simulink model "IEEE_13_BUS_Radial"  (R2021b)
settings: Solver=VariableStepAuto  StartTime=0.0  StopTime=48  RelTol=1e-3
undefined symbols (not defined in the file or in its folder): f611, f632, f633, f634, f645, f646, f650, f652, f671, f675, f680, f684, f692
libraries: simulink x416, slpidlib x13
(part 5 of 7)

== system IEEE_13_BUS_Radial/f692/PCU ==
  m : Inport
  setup : Inport  Port=2
  Psp : Inport  Port=3
  Bus Creator : BusCreator  Inputs=1
  Demux : Demux  Outputs=[1 -1]
  Mux2 : Mux  Inputs=16
  PID Controller : slpidlib/PID Controller  Controller=PID  Form=Parallel  TimeDomain=Continuous-time  UseExternalTs=off  SampleTime=-1  IntegratorMethod=Forward Euler  FilterMethod=Forward Euler  ControllerParametersSource=internal  P=80  I=20  D=10  UseFilter=on  N=100  TunerSelectOption=Transfer Function Based (PID Tuner App)  InitialConditionSource=internal  InitialConditionForIntegrator=0  InitialConditionForFilter=0  DifferentiatorICPrevScaledInput=0  ExternalReset=none  TrackingMode=off  Kt=1  LimitOutput=off  SatLimitsSource=internal  UpperSaturationLimit=inf  LowerSaturationLimit=-inf  LinearizeAsGain=on  AntiWindupMode=none  Kb=1  POutMin=[]  POutMax=[]  IOutMin=[]  IOutMax=[]  DOutMin=[]  DOutMax=[]  NOutMin=[]  NOutMax=[]  SumOutMin=[]  SumOutMax=[]  SaturationOutMin=[]  SaturationOutMax=[]  PParamMin=[]  PParamMax=[]  IParamMin=[]  IParamMax=[]  DParamMin=[]  DParamMax=[]  NParamMin=[]  NParamMax=[]  KbParamMin=[]  KbParamMax=[]  KtParamMin=[]  KtParamMax=[]  KbOutMin=[]  KbOutMax=[]  KtOutMin=[]  KtOutMax=[]  IntegratorOutMin=[]  IntegratorOutMax=[]  FilterOutMin=[]  FilterOutMax=[]  SumI1OutMin=[]  SumI1OutMax=[]  SumI2OutMin=[]  SumI2OutMax=[]  SumI3OutMin=[]  SumI3OutMax=[]  SumI4OutMin=[]  SumI4OutMax=[]  SumDOutMin=[]  SumDOutMax=[]  DifferentiatorOutMin=[]  DifferentiatorOutMax=[]  FilterDiffOutCoefMin=[]  FilterDiffOutCoefMax=[]  ReciprocalOutMin=[]  ReciprocalOutMax=[]  SumDenOutMin=[]  SumDenOutMax=[]  SumNumOutMin=[]  SumNumOutMax=[]  DivideOutMin=[]  DivideOutMax=[]  UdiffTsProdOutMin=[]  UdiffTsProdOutMax=[]  NTsProdOutMin=[]  NTsProdOutMax=[]  UintegralTsProdOutMin=[]  UintegralTsProdOutMax=[]  UngainTsProdOutMin=[]  UngainTsProdOutMax=[]  IntegratorContinuousStateAttributes=''  IntegratorStateMustResolveToSignalObject=off  IntegratorRTWStateStorageClass=Auto  FilterContinuousStateAttributes=''  FilterStateMustResolveToSignalObject=off  FilterRTWStateStorageClass=Auto  ParallelPVariant=InternalParameters  IdealPVariant=Disabled  IVariant=InternalParameters  DVariant=InternalParameters  IntegratorVariant=Continuous  SatVariant=Disabled  AWVariant=Passthrough  PCopyVariant=Disabled  TRVariant=Disabled  FdbkBlocksVariant=Forward  IdealPFdbkVariant=Disabled  SatFdbkVariant=Disabled  DerivativeFilterVariant=ContFilter  NVariant=InternalParameters  NCopyVariant=Disabled  FilterICVariant=InternalICsFilter  IntegratorICVariant=InternalICs  ExternalResetVariant=Disabled  TRSumVariant=Passthrough  SumFdbkVariant=Disabled  SumVariant=Sum_PID  TsampFilterVariant=InternalTs  TsampNgainVariant=Passthrough  TsampIntegralVariant=Passthrough  ExternalSaturationOutDataTypeStr=Inherit: Same as second input
  Sum : Sum  Inputs=+-
  Terminator : Terminator
  Terminator1 : Terminator
  sPCC : Constant  Value=0
  sPoLC{1,3..16} (15 alike) : Constant  Value=0
  sPoLC2 : Constant
  PCCctrl : Outport  VectorParamsAs1DForOutWhenUnconnected=off
  PoLCctrl : Outport  Port=2  VectorParamsAs1DForOutWhenUnconnected=off
  DEVctrl : Outport  Port=3  VectorParamsAs1DForOutWhenUnconnected=off
  wires:
  sPoLC8/1 -> Mux2/8
  sPoLC11/1 -> Mux2/11
  sPoLC4/1 -> Mux2/4
  sPoLC16/1 -> Mux2/16
  sPoLC14/1 -> Mux2/14
  sPoLC10/1 -> Mux2/10
  sPoLC12/1 -> Mux2/12
  sPoLC1/1 -> Mux2/1
  sPoLC15/1 -> Mux2/15
  sPoLC6/1 -> Mux2/6
  sPoLC13/1 -> Mux2/13
  sPoLC7/1 -> Mux2/7
  sPoLC9/1 -> Mux2/9
  sPoLC2/1 -> Mux2/2
  sPoLC3/1 -> Mux2/3
  sPoLC5/1 -> Mux2/5
  Mux2/1 -> PoLCctrl/1
  sPCC/1 -> PCCctrl/1
  setup/1 -> Terminator/1
  Psp/1 -> Sum/1
  Bus Creator/1 -> DEVctrl/1
  m/1 -> Demux/1
  Demux/1 -> Sum/2
  Sum/1 -> PID Controller/1
  PID Controller/1 -> Bus Creator/1  "pidCV"
  Demux/2 -> Terminator1/1

== system IEEE_13_BUS_Radial/f692/SYSTEM_INTERFACE ==
  ctrl : Inport
  devices : Inport  Port=2
  e_PoLC1 : Inport  Port=3
  e_PoLC2 : Inport  Port=4
  e_PoLC3 : Inport  Port=5
  e_PoLC4 : Inport  Port=6
  e_PoLC5 : Inport  Port=7
  e_PoLC6 : Inport  Port=8
  e_PoLC7 : Inport  Port=9
  e_PoLC8 : Inport  Port=10
  e_PoLC9 : Inport  Port=11
  e_PoLC10 : Inport  Port=12
  e_PoLC11 : Inport  Port=13
  e_PoLC12 : Inport  Port=14
  e_PoLC13 : Inport  Port=15
  e_PoLC14 : Inport  Port=16
  e_PoLC15 : Inport  Port=17
  e_PoLC16 : Inport  Port=18
  Demux : Demux  Outputs=16
  Demux1 : Demux  Outputs=16
  S PoLC{1..16} (16 alike) : Switch  Criteria=u2 > Threshold
  PoLC1 : Outport  VectorParamsAs1DForOutWhenUnconnected=off
  PoLC2 : Outport  Port=2  VectorParamsAs1DForOutWhenUnconnected=off
  PoLC3 : Outport  Port=3  VectorParamsAs1DForOutWhenUnconnected=off
  PoLC4 : Outport  Port=4  VectorParamsAs1DForOutWhenUnconnected=off
  PoLC5 : Outport  Port=5  VectorParamsAs1DForOutWhenUnconnected=off
  PoLC6 : Outport  Port=6  VectorParamsAs1DForOutWhenUnconnected=off
  PoLC7 : Outport  Port=7  VectorParamsAs1DForOutWhenUnconnected=off
  PoLC8 : Outport  Port=8  VectorParamsAs1DForOutWhenUnconnected=off
  PoLC9 : Outport  Port=9  VectorParamsAs1DForOutWhenUnconnected=off
  PoLC10 : Outport  Port=10  VectorParamsAs1DForOutWhenUnconnected=off
  PoLC11 : Outport  Port=11  VectorParamsAs1DForOutWhenUnconnected=off
  PoLC12 : Outport  Port=12  VectorParamsAs1DForOutWhenUnconnected=off
  PoLC13 : Outport  Port=13  VectorParamsAs1DForOutWhenUnconnected=off
  PoLC14 : Outport  Port=14  VectorParamsAs1DForOutWhenUnconnected=off
  PoLC15 : Outport  Port=15  VectorParamsAs1DForOutWhenUnconnected=off
  PoLC16 : Outport  Port=16  VectorParamsAs1DForOutWhenUnconnected=off
  wires:
  S PoLC9/1 -> PoLC9/1
  e_PoLC4/1 -> S PoLC4/3
  e_PoLC11/1 -> S PoLC11/3
  S PoLC16/1 -> PoLC16/1
  e_PoLC8/1 -> S PoLC8/3
  S PoLC6/1 -> PoLC6/1
  e_PoLC7/1 -> S PoLC7/3
  S PoLC13/1 -> PoLC13/1
  e_PoLC5/1 -> S PoLC5/3
  S PoLC10/1 -> PoLC10/1
  e_PoLC9/1 -> S PoLC9/3
  e_PoLC12/1 -> S PoLC12/3
  e_PoLC6/1 -> S PoLC6/3
  S PoLC15/1 -> PoLC15/1
  S PoLC1/1 -> PoLC1/1
  S PoLC12/1 -> PoLC12/1
  S PoLC11/1 -> PoLC11/1
  e_PoLC14/1 -> S PoLC14/3
  e_PoLC10/1 -> S PoLC10/3
  S PoLC5/1 -> PoLC5/1
  e_PoLC1/1 -> S PoLC1/3
  e_PoLC15/1 -> S PoLC15/3
  e_PoLC16/1 -> S PoLC16/3
  S PoLC7/1 -> PoLC7/1
  e_PoLC3/1 -> S PoLC3/3
  e_PoLC13/1 -> S PoLC13/3
  S PoLC8/1 -> PoLC8/1
  e_PoLC2/1 -> S PoLC2/3
  S PoLC4/1 -> PoLC4/1
  S PoLC2/1 -> PoLC2/1
  S PoLC14/1 -> PoLC14/1
  S PoLC3/1 -> PoLC3/1
  ctrl/1 -> Demux/1
  Demux/1 -> S PoLC1/2
  Demux/2 -> S PoLC2/2
  Demux/3 -> S PoLC3/2
  Demux/4 -> S PoLC4/2
  Demux/5 -> S PoLC5/2
  Demux/6 -> S PoLC6/2
  Demux/7 -> S PoLC7/2
  Demux/8 -> S PoLC8/2
  Demux/9 -> S PoLC9/2
  Demux/10 -> S PoLC10/2
  Demux/11 -> S PoLC11/2
  Demux/12 -> S PoLC12/2
  Demux/13 -> S PoLC13/2
  Demux/14 -> S PoLC14/2
  Demux/15 -> S PoLC15/2
  Demux/16 -> S PoLC16/2
  devices/1 -> Demux1/1
  Demux1/1 -> S PoLC1/1
  Demux1/2 -> S PoLC2/1
  Demux1/3 -> S PoLC3/1
  Demux1/4 -> S PoLC4/1
  Demux1/5 -> S PoLC5/1
  Demux1/6 -> S PoLC6/1
  Demux1/7 -> S PoLC7/1
  Demux1/8 -> S PoLC8/1
  Demux1/9 -> S PoLC9/1
  Demux1/10 -> S PoLC10/1
  Demux1/11 -> S PoLC11/1
  Demux1/12 -> S PoLC12/1
  Demux1/13 -> S PoLC13/1
  Demux1/14 -> S PoLC14/1
  Demux1/15 -> S PoLC15/1
  Demux1/16 -> S PoLC16/1

== system IEEE_13_BUS_Radial/f611/CONTROLLERS/lPoLC1 ==
  Sum : Sum  Inputs=|++
  base : simulink/Sources/Repeating Sequence Stair  OutValues=f611.PoLC1.l  tsamp=f611.PoLC1.ST  OutMin=[]  OutMax=[]  OutDataTypeStr=double  OutputDataTypeScalingMode=double  OutDataType=fixdt(0,8)  ConRadixGroup=Best Precision: Vector-wise  OutScaling=2^-12
  noise : simulink/Sources/Band-Limited White Noise  Cov=f611.PoLC1.Noise  Ts=f611.PoLC1.NoiseST  seed=f611.PoLC1.NoiseSD
  P : Outport  VectorParamsAs1DForOutWhenUnconnected=off
  wires:
  Sum/1 -> P/1
  noise/1 -> Sum/2
  base/1 -> Sum/1

== system IEEE_13_BUS_Radial/f611/CONTROLLERS/lPoLC10 ==
  Sum : Sum  Inputs=|++
  base : simulink/Sources/Repeating Sequence Stair  OutValues=f611.PoLC10.l  tsamp=f611.PoLC10.ST  OutMin=[]  OutMax=[]  OutDataTypeStr=double  OutputDataTypeScalingMode=double  OutDataType=fixdt(0,8)  ConRadixGroup=Best Precision: Vector-wise  OutScaling=2^-12
  noise : simulink/Sources/Band-Limited White Noise  Cov=f611.PoLC10.Noise  Ts=f611.PoLC10.NoiseST  seed=f611.PoLC10.NoiseSD
  P : Outport  VectorParamsAs1DForOutWhenUnconnected=off
  wires:
  Sum/1 -> P/1
  noise/1 -> Sum/2
  base/1 -> Sum/1

== system IEEE_13_BUS_Radial/f611/CONTROLLERS/lPoLC11 ==
  Sum : Sum  Inputs=|++
  base : simulink/Sources/Repeating Sequence Stair  OutValues=f611.PoLC11.l  tsamp=f611.PoLC11.ST  OutMin=[]  OutMax=[]  OutDataTypeStr=double  OutputDataTypeScalingMode=double  OutDataType=fixdt(0,8)  ConRadixGroup=Best Precision: Vector-wise  OutScaling=2^-12
  noise : simulink/Sources/Band-Limited White Noise  Cov=f611.PoLC11.Noise  Ts=f611.PoLC11.NoiseST  seed=f611.PoLC11.NoiseSD
  P : Outport  VectorParamsAs1DForOutWhenUnconnected=off
  wires:
  Sum/1 -> P/1
  noise/1 -> Sum/2
  base/1 -> Sum/1

== system IEEE_13_BUS_Radial/f611/CONTROLLERS/lPoLC12 ==
  Sum : Sum  Inputs=|++
  base : simulink/Sources/Repeating Sequence Stair  OutValues=f611.PoLC12.l  tsamp=f611.PoLC12.ST  OutMin=[]  OutMax=[]  OutDataTypeStr=double  OutputDataTypeScalingMode=double  OutDataType=fixdt(0,8)  ConRadixGroup=Best Precision: Vector-wise  OutScaling=2^-12
  noise : simulink/Sources/Band-Limited White Noise  Cov=f611.PoLC12.Noise  Ts=f611.PoLC12.NoiseST  seed=f611.PoLC12.NoiseSD
  P : Outport  VectorParamsAs1DForOutWhenUnconnected=off
  wires:
  Sum/1 -> P/1
  noise/1 -> Sum/2
  base/1 -> Sum/1

== system IEEE_13_BUS_Radial/f611/CONTROLLERS/lPoLC13 ==
  Sum : Sum  Inputs=|++
  base : simulink/Sources/Repeating Sequence Stair  OutValues=f611.PoLC13.l  tsamp=f611.PoLC13.ST  OutMin=[]  OutMax=[]  OutDataTypeStr=double  OutputDataTypeScalingMode=double  OutDataType=fixdt(0,8)  ConRadixGroup=Best Precision: Vector-wise  OutScaling=2^-12
  noise : simulink/Sources/Band-Limited White Noise  Cov=f611.PoLC13.Noise  Ts=f611.PoLC13.NoiseST  seed=f611.PoLC13.NoiseSD
  P : Outport  VectorParamsAs1DForOutWhenUnconnected=off
  wires:
  Sum/1 -> P/1
  noise/1 -> Sum/2
  base/1 -> Sum/1

== system IEEE_13_BUS_Radial/f611/CONTROLLERS/lPoLC14 ==
  Sum : Sum  Inputs=|++
  base : simulink/Sources/Repeating Sequence Stair  OutValues=f611.PoLC14.l  tsamp=f611.PoLC14.ST  OutMin=[]  OutMax=[]  OutDataTypeStr=double  OutputDataTypeScalingMode=double  OutDataType=fixdt(0,8)  ConRadixGroup=Best Precision: Vector-wise  OutScaling=2^-12
  noise : simulink/Sources/Band-Limited White Noise  Cov=f611.PoLC14.Noise  Ts=f611.PoLC14.NoiseST  seed=f611.PoLC14.NoiseSD
  P : Outport  VectorParamsAs1DForOutWhenUnconnected=off
  wires:
  Sum/1 -> P/1
  noise/1 -> Sum/2
  base/1 -> Sum/1

== system IEEE_13_BUS_Radial/f611/CONTROLLERS/lPoLC15 ==
  Sum : Sum  Inputs=|++
  base : simulink/Sources/Repeating Sequence Stair  OutValues=f611.PoLC15.l  tsamp=f611.PoLC15.ST  OutMin=[]  OutMax=[]  OutDataTypeStr=double  OutputDataTypeScalingMode=double  OutDataType=fixdt(0,8)  ConRadixGroup=Best Precision: Vector-wise  OutScaling=2^-12
  noise : simulink/Sources/Band-Limited White Noise  Cov=f611.PoLC15.Noise  Ts=f611.PoLC15.NoiseST  seed=f611.PoLC15.NoiseSD
  P : Outport  VectorParamsAs1DForOutWhenUnconnected=off
  wires:
  Sum/1 -> P/1
  noise/1 -> Sum/2
  base/1 -> Sum/1

== system IEEE_13_BUS_Radial/f611/CONTROLLERS/lPoLC16 ==
  cv : Inport
  Sum : Sum  Inputs=|++
  Terminator : Terminator
  base : simulink/Sources/Repeating Sequence Stair  OutValues=f611.PoLC16.l  tsamp=f611.PoLC16.ST  OutMin=[]  OutMax=[]  OutDataTypeStr=double  OutputDataTypeScalingMode=double  OutDataType=fixdt(0,8)  ConRadixGroup=Best Precision: Vector-wise  OutScaling=2^-12
  noise : simulink/Sources/Band-Limited White Noise  Cov=f611.PoLC16.Noise  Ts=f611.PoLC16.NoiseST  seed=f611.PoLC16.NoiseSD
  P : Outport  VectorParamsAs1DForOutWhenUnconnected=off
  wires:
  Sum/1 -> Terminator/1
  noise/1 -> Sum/2
  base/1 -> Sum/1
  cv/1 -> P/1

== system IEEE_13_BUS_Radial/f611/CONTROLLERS/lPoLC2 ==
  Sum : Sum  Inputs=|++
  base : simulink/Sources/Repeating Sequence Stair  OutValues=f611.PoLC2.l  tsamp=f611.PoLC2.ST  OutMin=[]  OutMax=[]  OutDataTypeStr=double  OutputDataTypeScalingMode=double  OutDataType=fixdt(0,8)  ConRadixGroup=Best Precision: Vector-wise  OutScaling=2^-12
  noise : simulink/Sources/Band-Limited White Noise  Cov=f611.PoLC2.Noise  Ts=f611.PoLC2.NoiseST  seed=f611.PoLC2.NoiseSD
  P : Outport  VectorParamsAs1DForOutWhenUnconnected=off
  wires:
  Sum/1 -> P/1
  noise/1 -> Sum/2
  base/1 -> Sum/1

== system IEEE_13_BUS_Radial/f611/CONTROLLERS/lPoLC3 ==
  Sum : Sum  Inputs=|++
  base : simulink/Sources/Repeating Sequence Stair  OutValues=f611.PoLC3.l  tsamp=f611.PoLC3.ST  OutMin=[]  OutMax=[]  OutDataTypeStr=double  OutputDataTypeScalingMode=double  OutDataType=fixdt(0,8)  ConRadixGroup=Best Precision: Vector-wise  OutScaling=2^-12
  noise : simulink/Sources/Band-Limited White Noise  Cov=f611.PoLC3.Noise  Ts=f611.PoLC3.NoiseST  seed=f611.PoLC3.NoiseSD
  P : Outport  VectorParamsAs1DForOutWhenUnconnected=off
  wires:
  Sum/1 -> P/1
  noise/1 -> Sum/2
  base/1 -> Sum/1

== system IEEE_13_BUS_Radial/f611/CONTROLLERS/lPoLC4 ==
  Sum : Sum  Inputs=|++
  base : simulink/Sources/Repeating Sequence Stair  OutValues=f611.PoLC4.l  tsamp=f611.PoLC4.ST  OutMin=[]  OutMax=[]  OutDataTypeStr=double  OutputDataTypeScalingMode=double  OutDataType=fixdt(0,8)  ConRadixGroup=Best Precision: Vector-wise  OutScaling=2^-12
  noise : simulink/Sources/Band-Limited White Noise  Cov=f611.PoLC4.Noise  Ts=f611.PoLC4.NoiseST  seed=f611.PoLC4.NoiseSD
  P : Outport  VectorParamsAs1DForOutWhenUnconnected=off
  wires:
  Sum/1 -> P/1
  noise/1 -> Sum/2
  base/1 -> Sum/1

== system IEEE_13_BUS_Radial/f611/CONTROLLERS/lPoLC5 ==
  Sum : Sum  Inputs=|++
  base : simulink/Sources/Repeating Sequence Stair  OutValues=f611.PoLC5.l  tsamp=f611.PoLC5.ST  OutMin=[]  OutMax=[]  OutDataTypeStr=double  OutputDataTypeScalingMode=double  OutDataType=fixdt(0,8)  ConRadixGroup=Best Precision: Vector-wise  OutScaling=2^-12
  noise : simulink/Sources/Band-Limited White Noise  Cov=f611.PoLC5.Noise  Ts=f611.PoLC5.NoiseST  seed=f611.PoLC5.NoiseSD
  P : Outport  VectorParamsAs1DForOutWhenUnconnected=off
  wires:
  Sum/1 -> P/1
  noise/1 -> Sum/2
  base/1 -> Sum/1

== system IEEE_13_BUS_Radial/f611/CONTROLLERS/lPoLC6 ==
  Sum : Sum  Inputs=|++
  base : simulink/Sources/Repeating Sequence Stair  OutValues=f611.PoLC6.l  tsamp=f611.PoLC6.ST  OutMin=[]  OutMax=[]  OutDataTypeStr=double  OutputDataTypeScalingMode=double  OutDataType=fixdt(0,8)  ConRadixGroup=Best Precision: Vector-wise  OutScaling=2^-12
  noise : simulink/Sources/Band-Limited White Noise  Cov=f611.PoLC6.Noise  Ts=f611.PoLC6.NoiseST  seed=f611.PoLC6.NoiseSD
  P : Outport  VectorParamsAs1DForOutWhenUnconnected=off
  wires:
  Sum/1 -> P/1
  noise/1 -> Sum/2
  base/1 -> Sum/1

== system IEEE_13_BUS_Radial/f611/CONTROLLERS/lPoLC7 ==
  Sum : Sum  Inputs=|++
  base : simulink/Sources/Repeating Sequence Stair  OutValues=f611.PoLC7.l  tsamp=f611.PoLC7.ST  OutMin=[]  OutMax=[]  OutDataTypeStr=double  OutputDataTypeScalingMode=double  OutDataType=fixdt(0,8)  ConRadixGroup=Best Precision: Vector-wise  OutScaling=2^-12
  noise : simulink/Sources/Band-Limited White Noise  Cov=f611.PoLC7.Noise  Ts=f611.PoLC7.NoiseST  seed=f611.PoLC7.NoiseSD
  P : Outport  VectorParamsAs1DForOutWhenUnconnected=off
  wires:
  Sum/1 -> P/1
  noise/1 -> Sum/2
  base/1 -> Sum/1

== system IEEE_13_BUS_Radial/f611/CONTROLLERS/lPoLC8 ==
  Sum : Sum  Inputs=|++
  base : simulink/Sources/Repeating Sequence Stair  OutValues=f611.PoLC8.l  tsamp=f611.PoLC8.ST  OutMin=[]  OutMax=[]  OutDataTypeStr=double  OutputDataTypeScalingMode=double  OutDataType=fixdt(0,8)  ConRadixGroup=Best Precision: Vector-wise  OutScaling=2^-12
  noise : simulink/Sources/Band-Limited White Noise  Cov=f611.PoLC8.Noise  Ts=f611.PoLC8.NoiseST  seed=f611.PoLC8.NoiseSD
  P : Outport  VectorParamsAs1DForOutWhenUnconnected=off
  wires:
  Sum/1 -> P/1
  noise/1 -> Sum/2
  base/1 -> Sum/1

== system IEEE_13_BUS_Radial/f611/CONTROLLERS/lPoLC9 ==
  Sum : Sum  Inputs=|++
  base : simulink/Sources/Repeating Sequence Stair  OutValues=f611.PoLC9.l  tsamp=f611.PoLC9.ST  OutMin=[]  OutMax=[]  OutDataTypeStr=double  OutputDataTypeScalingMode=double  OutDataType=fixdt(0,8)  ConRadixGroup=Best Precision: Vector-wise  OutScaling=2^-12
  noise : simulink/Sources/Band-Limited White Noise  Cov=f611.PoLC9.Noise  Ts=f611.PoLC9.NoiseST  seed=f611.PoLC9.NoiseSD
  P : Outport  VectorParamsAs1DForOutWhenUnconnected=off
  wires:
  Sum/1 -> P/1
  noise/1 -> Sum/2
  base/1 -> Sum/1

== system IEEE_13_BUS_Radial/f611/OPERATIONS GATEWAY/Agent Communications ==
  Enable : EnablePort
  Constant : Constant  Value=0
  Out1 : Outport  VectorParamsAs1DForOutWhenUnconnected=off
  wires:
  Constant/1 -> Out1/1

== system IEEE_13_BUS_Radial/f632/CONTROLLERS/lPoLC1 ==
  Sum : Sum  Inputs=|++
  base : simulink/Sources/Repeating Sequence Stair  OutValues=f632.PoLC1.l  tsamp=f632.PoLC1.ST  OutMin=[]  OutMax=[]  OutDataTypeStr=double  OutputDataTypeScalingMode=double  OutDataType=fixdt(0,8)  ConRadixGroup=Best Precision: Vector-wise  OutScaling=2^-12
  noise : simulink/Sources/Band-Limited White Noise  Cov=f632.PoLC1.Noise  Ts=f632.PoLC1.NoiseST  seed=f632.PoLC1.NoiseSD
  P : Outport  VectorParamsAs1DForOutWhenUnconnected=off
  wires:
  base/1 -> Sum/1
  noise/1 -> Sum/2
  Sum/1 -> P/1

== system IEEE_13_BUS_Radial/f632/CONTROLLERS/lPoLC10 ==
  Sum : Sum  Inputs=|++
  base : simulink/Sources/Repeating Sequence Stair  OutValues=f632.PoLC10.l  tsamp=f632.PoLC10.ST  OutMin=[]  OutMax=[]  OutDataTypeStr=double  OutputDataTypeScalingMode=double  OutDataType=fixdt(0,8)  ConRadixGroup=Best Precision: Vector-wise  OutScaling=2^-12
  noise : simulink/Sources/Band-Limited White Noise  Cov=f632.PoLC10.Noise  Ts=f632.PoLC10.NoiseST  seed=f632.PoLC10.NoiseSD
  P : Outport  VectorParamsAs1DForOutWhenUnconnected=off
  wires:
  base/1 -> Sum/1
  noise/1 -> Sum/2
  Sum/1 -> P/1

== system IEEE_13_BUS_Radial/f632/CONTROLLERS/lPoLC11 ==
  Sum : Sum  Inputs=|++
  base : simulink/Sources/Repeating Sequence Stair  OutValues=f632.PoLC11.l  tsamp=f632.PoLC11.ST  OutMin=[]  OutMax=[]  OutDataTypeStr=double  OutputDataTypeScalingMode=double  OutDataType=fixdt(0,8)  ConRadixGroup=Best Precision: Vector-wise  OutScaling=2^-12
  noise : simulink/Sources/Band-Limited White Noise  Cov=f632.PoLC11.Noise  Ts=f632.PoLC11.NoiseST  seed=f632.PoLC11.NoiseSD
  P : Outport  VectorParamsAs1DForOutWhenUnconnected=off
  wires:
  base/1 -> Sum/1
  noise/1 -> Sum/2
  Sum/1 -> P/1

== system IEEE_13_BUS_Radial/f632/CONTROLLERS/lPoLC12 ==
  Sum : Sum  Inputs=|++
  base : simulink/Sources/Repeating Sequence Stair  OutValues=f632.PoLC12.l  tsamp=f632.PoLC12.ST  OutMin=[]  OutMax=[]  OutDataTypeStr=double  OutputDataTypeScalingMode=double  OutDataType=fixdt(0,8)  ConRadixGroup=Best Precision: Vector-wise  OutScaling=2^-12
  noise : simulink/Sources/Band-Limited White Noise  Cov=f632.PoLC12.Noise  Ts=f632.PoLC12.NoiseST  seed=f632.PoLC12.NoiseSD
  P : Outport  VectorParamsAs1DForOutWhenUnconnected=off
  wires:
  base/1 -> Sum/1
  noise/1 -> Sum/2
  Sum/1 -> P/1

== system IEEE_13_BUS_Radial/f632/CONTROLLERS/lPoLC13 ==
  Sum : Sum  Inputs=|++
  base : simulink/Sources/Repeating Sequence Stair  OutValues=f632.PoLC13.l  tsamp=f632.PoLC13.ST  OutMin=[]  OutMax=[]  OutDataTypeStr=double  OutputDataTypeScalingMode=double  OutDataType=fixdt(0,8)  ConRadixGroup=Best Precision: Vector-wise  OutScaling=2^-12
  noise : simulink/Sources/Band-Limited White Noise  Cov=f632.PoLC13.Noise  Ts=f632.PoLC13.NoiseST  seed=f632.PoLC13.NoiseSD
  P : Outport  VectorParamsAs1DForOutWhenUnconnected=off
  wires:
  base/1 -> Sum/1
  noise/1 -> Sum/2
  Sum/1 -> P/1

== system IEEE_13_BUS_Radial/f632/CONTROLLERS/lPoLC14 ==
  Sum : Sum  Inputs=|++
  base : simulink/Sources/Repeating Sequence Stair  OutValues=f632.PoLC14.l  tsamp=f632.PoLC14.ST  OutMin=[]  OutMax=[]  OutDataTypeStr=double  OutputDataTypeScalingMode=double  OutDataType=fixdt(0,8)  ConRadixGroup=Best Precision: Vector-wise  OutScaling=2^-12
  noise : simulink/Sources/Band-Limited White Noise  Cov=f632.PoLC14.Noise  Ts=f632.PoLC14.NoiseST  seed=f632.PoLC14.NoiseSD
  P : Outport  VectorParamsAs1DForOutWhenUnconnected=off
  wires:
  base/1 -> Sum/1
  noise/1 -> Sum/2
  Sum/1 -> P/1

== system IEEE_13_BUS_Radial/f632/CONTROLLERS/lPoLC15 ==
  Sum : Sum  Inputs=|++
  base : simulink/Sources/Repeating Sequence Stair  OutValues=f632.PoLC15.l  tsamp=f632.PoLC15.ST  OutMin=[]  OutMax=[]  OutDataTypeStr=double  OutputDataTypeScalingMode=double  OutDataType=fixdt(0,8)  ConRadixGroup=Best Precision: Vector-wise  OutScaling=2^-12
  noise : simulink/Sources/Band-Limited White Noise  Cov=f632.PoLC15.Noise  Ts=f632.PoLC15.NoiseST  seed=f632.PoLC15.NoiseSD
  P : Outport  VectorParamsAs1DForOutWhenUnconnected=off
  wires:
  base/1 -> Sum/1
  noise/1 -> Sum/2
  Sum/1 -> P/1

== system IEEE_13_BUS_Radial/f632/CONTROLLERS/lPoLC16 ==
  cv : Inport
  Sum : Sum  Inputs=|++
  Terminator : Terminator
  base : simulink/Sources/Repeating Sequence Stair  OutValues=f632.PoLC16.l  tsamp=f632.PoLC16.ST  OutMin=[]  OutMax=[]  OutDataTypeStr=double  OutputDataTypeScalingMode=double  OutDataType=fixdt(0,8)  ConRadixGroup=Best Precision: Vector-wise  OutScaling=2^-12
  noise : simulink/Sources/Band-Limited White Noise  Cov=f632.PoLC16.Noise  Ts=f632.PoLC16.NoiseST  seed=f632.PoLC16.NoiseSD
  P : Outport  VectorParamsAs1DForOutWhenUnconnected=off
  wires:
  cv/1 -> P/1
  base/1 -> Sum/1
  noise/1 -> Sum/2
  Sum/1 -> Terminator/1

== system IEEE_13_BUS_Radial/f632/CONTROLLERS/lPoLC2 ==
  Sum : Sum  Inputs=|++
  base : simulink/Sources/Repeating Sequence Stair  OutValues=f632.PoLC2.l  tsamp=f632.PoLC2.ST  OutMin=[]  OutMax=[]  OutDataTypeStr=double  OutputDataTypeScalingMode=double  OutDataType=fixdt(0,8)  ConRadixGroup=Best Precision: Vector-wise  OutScaling=2^-12
  noise : simulink/Sources/Band-Limited White Noise  Cov=f632.PoLC2.Noise  Ts=f632.PoLC2.NoiseST  seed=f632.PoLC2.NoiseSD
  P : Outport  VectorParamsAs1DForOutWhenUnconnected=off
  wires:
  base/1 -> Sum/1
  noise/1 -> Sum/2
  Sum/1 -> P/1

== system IEEE_13_BUS_Radial/f632/CONTROLLERS/lPoLC3 ==
  Sum : Sum  Inputs=|++
  base : simulink/Sources/Repeating Sequence Stair  OutValues=f632.PoLC3.l  tsamp=f632.PoLC3.ST  OutMin=[]  OutMax=[]  OutDataTypeStr=double  OutputDataTypeScalingMode=double  OutDataType=fixdt(0,8)  ConRadixGroup=Best Precision: Vector-wise  OutScaling=2^-12
  noise : simulink/Sources/Band-Limited White Noise  Cov=f632.PoLC3.Noise  Ts=f632.PoLC3.NoiseST  seed=f632.PoLC3.NoiseSD
  P : Outport  VectorParamsAs1DForOutWhenUnconnected=off
  wires:
  base/1 -> Sum/1
  noise/1 -> Sum/2
  Sum/1 -> P/1

== system IEEE_13_BUS_Radial/f632/CONTROLLERS/lPoLC4 ==
  Sum : Sum  Inputs=|++
  base : simulink/Sources/Repeating Sequence Stair  OutValues=f632.PoLC4.l  tsamp=f632.PoLC4.ST  OutMin=[]  OutMax=[]  OutDataTypeStr=double  OutputDataTypeScalingMode=double  OutDataType=fixdt(0,8)  ConRadixGroup=Best Precision: Vector-wise  OutScaling=2^-12
  noise : simulink/Sources/Band-Limited White Noise  Cov=f632.PoLC4.Noise  Ts=f632.PoLC4.NoiseST  seed=f632.PoLC4.NoiseSD
  P : Outport  VectorParamsAs1DForOutWhenUnconnected=off
  wires:
  base/1 -> Sum/1
  noise/1 -> Sum/2
  Sum/1 -> P/1

== system IEEE_13_BUS_Radial/f632/CONTROLLERS/lPoLC5 ==
  Sum : Sum  Inputs=|++
  base : simulink/Sources/Repeating Sequence Stair  OutValues=f632.PoLC5.l  tsamp=f632.PoLC5.ST  OutMin=[]  OutMax=[]  OutDataTypeStr=double  OutputDataTypeScalingMode=double  OutDataType=fixdt(0,8)  ConRadixGroup=Best Precision: Vector-wise  OutScaling=2^-12
  noise : simulink/Sources/Band-Limited White Noise  Cov=f632.PoLC5.Noise  Ts=f632.PoLC5.NoiseST  seed=f632.PoLC5.NoiseSD
  P : Outport  VectorParamsAs1DForOutWhenUnconnected=off
  wires:
  base/1 -> Sum/1
  noise/1 -> Sum/2
  Sum/1 -> P/1

== system IEEE_13_BUS_Radial/f632/CONTROLLERS/lPoLC6 ==
  Sum : Sum  Inputs=|++
  base : simulink/Sources/Repeating Sequence Stair  OutValues=f632.PoLC6.l  tsamp=f632.PoLC6.ST  OutMin=[]  OutMax=[]  OutDataTypeStr=double  OutputDataTypeScalingMode=double  OutDataType=fixdt(0,8)  ConRadixGroup=Best Precision: Vector-wise  OutScaling=2^-12
  noise : simulink/Sources/Band-Limited White Noise  Cov=f632.PoLC6.Noise  Ts=f632.PoLC6.NoiseST  seed=f632.PoLC6.NoiseSD
  P : Outport  VectorParamsAs1DForOutWhenUnconnected=off
  wires:
  base/1 -> Sum/1
  noise/1 -> Sum/2
  Sum/1 -> P/1

== system IEEE_13_BUS_Radial/f632/CONTROLLERS/lPoLC7 ==
  Sum : Sum  Inputs=|++
  base : simulink/Sources/Repeating Sequence Stair  OutValues=f632.PoLC7.l  tsamp=f632.PoLC7.ST  OutMin=[]  OutMax=[]  OutDataTypeStr=double  OutputDataTypeScalingMode=double  OutDataType=fixdt(0,8)  ConRadixGroup=Best Precision: Vector-wise  OutScaling=2^-12
  noise : simulink/Sources/Band-Limited White Noise  Cov=f632.PoLC7.Noise  Ts=f632.PoLC7.NoiseST  seed=f632.PoLC7.NoiseSD
  P : Outport  VectorParamsAs1DForOutWhenUnconnected=off
  wires:
  base/1 -> Sum/1
  noise/1 -> Sum/2
  Sum/1 -> P/1

== system IEEE_13_BUS_Radial/f632/CONTROLLERS/lPoLC8 ==
  Sum : Sum  Inputs=|++
  base : simulink/Sources/Repeating Sequence Stair  OutValues=f632.PoLC8.l  tsamp=f632.PoLC8.ST  OutMin=[]  OutMax=[]  OutDataTypeStr=double  OutputDataTypeScalingMode=double  OutDataType=fixdt(0,8)  ConRadixGroup=Best Precision: Vector-wise  OutScaling=2^-12
  noise : simulink/Sources/Band-Limited White Noise  Cov=f632.PoLC8.Noise  Ts=f632.PoLC8.NoiseST  seed=f632.PoLC8.NoiseSD
  P : Outport  VectorParamsAs1DForOutWhenUnconnected=off
  wires:
  base/1 -> Sum/1
  noise/1 -> Sum/2
  Sum/1 -> P/1

== system IEEE_13_BUS_Radial/f632/CONTROLLERS/lPoLC9 ==
  Sum : Sum  Inputs=|++
  base : simulink/Sources/Repeating Sequence Stair  OutValues=f632.PoLC9.l  tsamp=f632.PoLC9.ST  OutMin=[]  OutMax=[]  OutDataTypeStr=double  OutputDataTypeScalingMode=double  OutDataType=fixdt(0,8)  ConRadixGroup=Best Precision: Vector-wise  OutScaling=2^-12
  noise : simulink/Sources/Band-Limited White Noise  Cov=f632.PoLC9.Noise  Ts=f632.PoLC9.NoiseST  seed=f632.PoLC9.NoiseSD
  P : Outport  VectorParamsAs1DForOutWhenUnconnected=off
  wires:
  base/1 -> Sum/1
  noise/1 -> Sum/2
  Sum/1 -> P/1

== system IEEE_13_BUS_Radial/f632/OPERATIONS GATEWAY/Agent Communications ==
  Enable : EnablePort
  Constant : Constant  Value=0
  Out1 : Outport  VectorParamsAs1DForOutWhenUnconnected=off
  wires:
  Constant/1 -> Out1/1

== system IEEE_13_BUS_Radial/f633/CONTROLLERS/lPoLC1 ==
  Sum : Sum  Inputs=|++
  base : simulink/Sources/Repeating Sequence Stair  OutValues=f633.PoLC1.l  tsamp=f633.PoLC1.ST  OutMin=[]  OutMax=[]  OutDataTypeStr=double  OutputDataTypeScalingMode=double  OutDataType=fixdt(0,8)  ConRadixGroup=Best Precision: Vector-wise  OutScaling=2^-12
  noise : simulink/Sources/Band-Limited White Noise  Cov=f633.PoLC1.Noise  Ts=f633.PoLC1.NoiseST  seed=f633.PoLC1.NoiseSD
  P : Outport  VectorParamsAs1DForOutWhenUnconnected=off
  wires:
  Sum/1 -> P/1
  noise/1 -> Sum/2
  base/1 -> Sum/1

== system IEEE_13_BUS_Radial/f633/CONTROLLERS/lPoLC10 ==
  Sum : Sum  Inputs=|++
  base : simulink/Sources/Repeating Sequence Stair  OutValues=f633.PoLC10.l  tsamp=f633.PoLC10.ST  OutMin=[]  OutMax=[]  OutDataTypeStr=double  OutputDataTypeScalingMode=double  OutDataType=fixdt(0,8)  ConRadixGroup=Best Precision: Vector-wise  OutScaling=2^-12
  noise : simulink/Sources/Band-Limited White Noise  Cov=f633.PoLC10.Noise  Ts=f633.PoLC10.NoiseST  seed=f633.PoLC10.NoiseSD
  P : Outport  VectorParamsAs1DForOutWhenUnconnected=off
  wires:
  Sum/1 -> P/1
  noise/1 -> Sum/2
  base/1 -> Sum/1

== system IEEE_13_BUS_Radial/f633/CONTROLLERS/lPoLC11 ==
  Sum : Sum  Inputs=|++
  base : simulink/Sources/Repeating Sequence Stair  OutValues=f633.PoLC11.l  tsamp=f633.PoLC11.ST  OutMin=[]  OutMax=[]  OutDataTypeStr=double  OutputDataTypeScalingMode=double  OutDataType=fixdt(0,8)  ConRadixGroup=Best Precision: Vector-wise  OutScaling=2^-12
  noise : simulink/Sources/Band-Limited White Noise  Cov=f633.PoLC11.Noise  Ts=f633.PoLC11.NoiseST  seed=f633.PoLC11.NoiseSD
  P : Outport  VectorParamsAs1DForOutWhenUnconnected=off
  wires:
  Sum/1 -> P/1
  noise/1 -> Sum/2
  base/1 -> Sum/1

== system IEEE_13_BUS_Radial/f633/CONTROLLERS/lPoLC12 ==
  Sum : Sum  Inputs=|++
  base : simulink/Sources/Repeating Sequence Stair  OutValues=f633.PoLC12.l  tsamp=f633.PoLC12.ST  OutMin=[]  OutMax=[]  OutDataTypeStr=double  OutputDataTypeScalingMode=double  OutDataType=fixdt(0,8)  ConRadixGroup=Best Precision: Vector-wise  OutScaling=2^-12
  noise : simulink/Sources/Band-Limited White Noise  Cov=f633.PoLC12.Noise  Ts=f633.PoLC12.NoiseST  seed=f633.PoLC12.NoiseSD
  P : Outport  VectorParamsAs1DForOutWhenUnconnected=off
  wires:
  Sum/1 -> P/1
  noise/1 -> Sum/2
  base/1 -> Sum/1

== system IEEE_13_BUS_Radial/f633/CONTROLLERS/lPoLC13 ==
  Sum : Sum  Inputs=|++
  base : simulink/Sources/Repeating Sequence Stair  OutValues=f633.PoLC13.l  tsamp=f633.PoLC13.ST  OutMin=[]  OutMax=[]  OutDataTypeStr=double  OutputDataTypeScalingMode=double  OutDataType=fixdt(0,8)  ConRadixGroup=Best Precision: Vector-wise  OutScaling=2^-12
  noise : simulink/Sources/Band-Limited White Noise  Cov=f633.PoLC13.Noise  Ts=f633.PoLC13.NoiseST  seed=f633.PoLC13.NoiseSD
  P : Outport  VectorParamsAs1DForOutWhenUnconnected=off
  wires:
  Sum/1 -> P/1
  noise/1 -> Sum/2
  base/1 -> Sum/1

== system IEEE_13_BUS_Radial/f633/CONTROLLERS/lPoLC14 ==
  Sum : Sum  Inputs=|++
  base : simulink/Sources/Repeating Sequence Stair  OutValues=f633.PoLC14.l  tsamp=f633.PoLC14.ST  OutMin=[]  OutMax=[]  OutDataTypeStr=double  OutputDataTypeScalingMode=double  OutDataType=fixdt(0,8)  ConRadixGroup=Best Precision: Vector-wise  OutScaling=2^-12
  noise : simulink/Sources/Band-Limited White Noise  Cov=f633.PoLC14.Noise  Ts=f633.PoLC14.NoiseST  seed=f633.PoLC14.NoiseSD
  P : Outport  VectorParamsAs1DForOutWhenUnconnected=off
  wires:
  Sum/1 -> P/1
  noise/1 -> Sum/2
  base/1 -> Sum/1

== system IEEE_13_BUS_Radial/f633/CONTROLLERS/lPoLC15 ==
  Sum : Sum  Inputs=|++
  base : simulink/Sources/Repeating Sequence Stair  OutValues=f633.PoLC15.l  tsamp=f633.PoLC15.ST  OutMin=[]  OutMax=[]  OutDataTypeStr=double  OutputDataTypeScalingMode=double  OutDataType=fixdt(0,8)  ConRadixGroup=Best Precision: Vector-wise  OutScaling=2^-12
  noise : simulink/Sources/Band-Limited White Noise  Cov=f633.PoLC15.Noise  Ts=f633.PoLC15.NoiseST  seed=f633.PoLC15.NoiseSD
  P : Outport  VectorParamsAs1DForOutWhenUnconnected=off
  wires:
  Sum/1 -> P/1
  noise/1 -> Sum/2
  base/1 -> Sum/1

== system IEEE_13_BUS_Radial/f633/CONTROLLERS/lPoLC16 ==
  cv : Inport
  Sum : Sum  Inputs=|++
  Terminator : Terminator
  base : simulink/Sources/Repeating Sequence Stair  OutValues=f633.PoLC16.l  tsamp=f633.PoLC16.ST  OutMin=[]  OutMax=[]  OutDataTypeStr=double  OutputDataTypeScalingMode=double  OutDataType=fixdt(0,8)  ConRadixGroup=Best Precision: Vector-wise  OutScaling=2^-12
  noise : simulink/Sources/Band-Limited White Noise  Cov=f633.PoLC16.Noise  Ts=f633.PoLC16.NoiseST  seed=f633.PoLC16.NoiseSD
  P : Outport  VectorParamsAs1DForOutWhenUnconnected=off
  wires:
  Sum/1 -> Terminator/1
  noise/1 -> Sum/2
  base/1 -> Sum/1
  cv/1 -> P/1

== system IEEE_13_BUS_Radial/f633/CONTROLLERS/lPoLC2 ==
  Sum : Sum  Inputs=|++
  base : simulink/Sources/Repeating Sequence Stair  OutValues=f633.PoLC2.l  tsamp=f633.PoLC2.ST  OutMin=[]  OutMax=[]  OutDataTypeStr=double  OutputDataTypeScalingMode=double  OutDataType=fixdt(0,8)  ConRadixGroup=Best Precision: Vector-wise  OutScaling=2^-12
  noise : simulink/Sources/Band-Limited White Noise  Cov=f633.PoLC2.Noise  Ts=f633.PoLC2.NoiseST  seed=f633.PoLC2.NoiseSD
  P : Outport  VectorParamsAs1DForOutWhenUnconnected=off
  wires:
  Sum/1 -> P/1
  noise/1 -> Sum/2
  base/1 -> Sum/1

== system IEEE_13_BUS_Radial/f633/CONTROLLERS/lPoLC3 ==
  Sum : Sum  Inputs=|++
  base : simulink/Sources/Repeating Sequence Stair  OutValues=f633.PoLC3.l  tsamp=f633.PoLC3.ST  OutMin=[]  OutMax=[]  OutDataTypeStr=double  OutputDataTypeScalingMode=double  OutDataType=fixdt(0,8)  ConRadixGroup=Best Precision: Vector-wise  OutScaling=2^-12
  noise : simulink/Sources/Band-Limited White Noise  Cov=f633.PoLC3.Noise  Ts=f633.PoLC3.NoiseST  seed=f633.PoLC3.NoiseSD
  P : Outport  VectorParamsAs1DForOutWhenUnconnected=off
  wires:
  Sum/1 -> P/1
  noise/1 -> Sum/2
  base/1 -> Sum/1

== system IEEE_13_BUS_Radial/f633/CONTROLLERS/lPoLC4 ==
  Sum : Sum  Inputs=|++
  base : simulink/Sources/Repeating Sequence Stair  OutValues=f633.PoLC4.l  tsamp=f633.PoLC4.ST  OutMin=[]  OutMax=[]  OutDataTypeStr=double  OutputDataTypeScalingMode=double  OutDataType=fixdt(0,8)  ConRadixGroup=Best Precision: Vector-wise  OutScaling=2^-12
  noise : simulink/Sources/Band-Limited White Noise  Cov=f633.PoLC4.Noise  Ts=f633.PoLC4.NoiseST  seed=f633.PoLC4.NoiseSD
  P : Outport  VectorParamsAs1DForOutWhenUnconnected=off
  wires:
  Sum/1 -> P/1
  noise/1 -> Sum/2
  base/1 -> Sum/1

== system IEEE_13_BUS_Radial/f633/CONTROLLERS/lPoLC5 ==
  Sum : Sum  Inputs=|++
  base : simulink/Sources/Repeating Sequence Stair  OutValues=f633.PoLC5.l  tsamp=f633.PoLC5.ST  OutMin=[]  OutMax=[]  OutDataTypeStr=double  OutputDataTypeScalingMode=double  OutDataType=fixdt(0,8)  ConRadixGroup=Best Precision: Vector-wise  OutScaling=2^-12
  noise : simulink/Sources/Band-Limited White Noise  Cov=f633.PoLC5.Noise  Ts=f633.PoLC5.NoiseST  seed=f633.PoLC5.NoiseSD
  P : Outport  VectorParamsAs1DForOutWhenUnconnected=off
  wires:
  Sum/1 -> P/1
  noise/1 -> Sum/2
  base/1 -> Sum/1

== system IEEE_13_BUS_Radial/f633/CONTROLLERS/lPoLC6 ==
  Sum : Sum  Inputs=|++
  base : simulink/Sources/Repeating Sequence Stair  OutValues=f633.PoLC6.l  tsamp=f633.PoLC6.ST  OutMin=[]  OutMax=[]  OutDataTypeStr=double  OutputDataTypeScalingMode=double  OutDataType=fixdt(0,8)  ConRadixGroup=Best Precision: Vector-wise  OutScaling=2^-12
  noise : simulink/Sources/Band-Limited White Noise  Cov=f633.PoLC6.Noise  Ts=f633.PoLC6.NoiseST  seed=f633.PoLC6.NoiseSD
  P : Outport  VectorParamsAs1DForOutWhenUnconnected=off
  wires:
  Sum/1 -> P/1
  noise/1 -> Sum/2
  base/1 -> Sum/1

== system IEEE_13_BUS_Radial/f633/CONTROLLERS/lPoLC7 ==
  Sum : Sum  Inputs=|++
  base : simulink/Sources/Repeating Sequence Stair  OutValues=f633.PoLC7.l  tsamp=f633.PoLC7.ST  OutMin=[]  OutMax=[]  OutDataTypeStr=double  OutputDataTypeScalingMode=double  OutDataType=fixdt(0,8)  ConRadixGroup=Best Precision: Vector-wise  OutScaling=2^-12
  noise : simulink/Sources/Band-Limited White Noise  Cov=f633.PoLC7.Noise  Ts=f633.PoLC7.NoiseST  seed=f633.PoLC7.NoiseSD
  P : Outport  VectorParamsAs1DForOutWhenUnconnected=off
  wires:
  Sum/1 -> P/1
  noise/1 -> Sum/2
  base/1 -> Sum/1

== system IEEE_13_BUS_Radial/f633/CONTROLLERS/lPoLC8 ==
  Sum : Sum  Inputs=|++
  base : simulink/Sources/Repeating Sequence Stair  OutValues=f633.PoLC8.l  tsamp=f633.PoLC8.ST  OutMin=[]  OutMax=[]  OutDataTypeStr=double  OutputDataTypeScalingMode=double  OutDataType=fixdt(0,8)  ConRadixGroup=Best Precision: Vector-wise  OutScaling=2^-12
  noise : simulink/Sources/Band-Limited White Noise  Cov=f633.PoLC8.Noise  Ts=f633.PoLC8.NoiseST  seed=f633.PoLC8.NoiseSD
  P : Outport  VectorParamsAs1DForOutWhenUnconnected=off
  wires:
  Sum/1 -> P/1
  noise/1 -> Sum/2
  base/1 -> Sum/1

== system IEEE_13_BUS_Radial/f633/CONTROLLERS/lPoLC9 ==
  Sum : Sum  Inputs=|++
  base : simulink/Sources/Repeating Sequence Stair  OutValues=f633.PoLC9.l  tsamp=f633.PoLC9.ST  OutMin=[]  OutMax=[]  OutDataTypeStr=double  OutputDataTypeScalingMode=double  OutDataType=fixdt(0,8)  ConRadixGroup=Best Precision: Vector-wise  OutScaling=2^-12
  noise : simulink/Sources/Band-Limited White Noise  Cov=f633.PoLC9.Noise  Ts=f633.PoLC9.NoiseST  seed=f633.PoLC9.NoiseSD
  P : Outport  VectorParamsAs1DForOutWhenUnconnected=off
  wires:
  Sum/1 -> P/1
  noise/1 -> Sum/2
  base/1 -> Sum/1

== system IEEE_13_BUS_Radial/f633/OPERATIONS GATEWAY/Agent Communications ==
  Enable : EnablePort
  Constant : Constant  Value=0
  Out1 : Outport  VectorParamsAs1DForOutWhenUnconnected=off
  wires:
  Constant/1 -> Out1/1

== system IEEE_13_BUS_Radial/f634/CONTROLLERS/lPoLC1 ==
  Sum : Sum  Inputs=|++
  base : simulink/Sources/Repeating Sequence Stair  OutValues=f634.PoLC1.l  tsamp=f634.PoLC1.ST  OutMin=[]  OutMax=[]  OutDataTypeStr=double  OutputDataTypeScalingMode=double  OutDataType=fixdt(0,8)  ConRadixGroup=Best Precision: Vector-wise  OutScaling=2^-12
  noise : simulink/Sources/Band-Limited White Noise  Cov=f634.PoLC1.Noise  Ts=f634.PoLC1.NoiseST  seed=f634.PoLC1.NoiseSD
  P : Outport  VectorParamsAs1DForOutWhenUnconnected=off
  wires:
  Sum/1 -> P/1
  noise/1 -> Sum/2
  base/1 -> Sum/1

== system IEEE_13_BUS_Radial/f634/CONTROLLERS/lPoLC10 ==
  Sum : Sum  Inputs=|++
  base : simulink/Sources/Repeating Sequence Stair  OutValues=f634.PoLC10.l  tsamp=f634.PoLC10.ST  OutMin=[]  OutMax=[]  OutDataTypeStr=double  OutputDataTypeScalingMode=double  OutDataType=fixdt(0,8)  ConRadixGroup=Best Precision: Vector-wise  OutScaling=2^-12
  noise : simulink/Sources/Band-Limited White Noise  Cov=f634.PoLC10.Noise  Ts=f634.PoLC10.NoiseST  seed=f634.PoLC10.NoiseSD
  P : Outport  VectorParamsAs1DForOutWhenUnconnected=off
  wires:
  Sum/1 -> P/1
  noise/1 -> Sum/2
  base/1 -> Sum/1

== system IEEE_13_BUS_Radial/f634/CONTROLLERS/lPoLC11 ==
  Sum : Sum  Inputs=|++
  base : simulink/Sources/Repeating Sequence Stair  OutValues=f634.PoLC11.l  tsamp=f634.PoLC11.ST  OutMin=[]  OutMax=[]  OutDataTypeStr=double  OutputDataTypeScalingMode=double  OutDataType=fixdt(0,8)  ConRadixGroup=Best Precision: Vector-wise  OutScaling=2^-12
  noise : simulink/Sources/Band-Limited White Noise  Cov=f634.PoLC11.Noise  Ts=f634.PoLC11.NoiseST  seed=f634.PoLC11.NoiseSD
  P : Outport  VectorParamsAs1DForOutWhenUnconnected=off
  wires:
  Sum/1 -> P/1
  noise/1 -> Sum/2
  base/1 -> Sum/1

== system IEEE_13_BUS_Radial/f634/CONTROLLERS/lPoLC12 ==
  Sum : Sum  Inputs=|++
  base : simulink/Sources/Repeating Sequence Stair  OutValues=f634.PoLC12.l  tsamp=f634.PoLC12.ST  OutMin=[]  OutMax=[]  OutDataTypeStr=double  OutputDataTypeScalingMode=double  OutDataType=fixdt(0,8)  ConRadixGroup=Best Precision: Vector-wise  OutScaling=2^-12
  noise : simulink/Sources/Band-Limited White Noise  Cov=f634.PoLC12.Noise  Ts=f634.PoLC12.NoiseST  seed=f634.PoLC12.NoiseSD
  P : Outport  VectorParamsAs1DForOutWhenUnconnected=off
  wires:
  Sum/1 -> P/1
  noise/1 -> Sum/2
  base/1 -> Sum/1

== system IEEE_13_BUS_Radial/f634/CONTROLLERS/lPoLC13 ==
  Sum : Sum  Inputs=|++
  base : simulink/Sources/Repeating Sequence Stair  OutValues=f634.PoLC13.l  tsamp=f634.PoLC13.ST  OutMin=[]  OutMax=[]  OutDataTypeStr=double  OutputDataTypeScalingMode=double  OutDataType=fixdt(0,8)  ConRadixGroup=Best Precision: Vector-wise  OutScaling=2^-12
  noise : simulink/Sources/Band-Limited White Noise  Cov=f634.PoLC13.Noise  Ts=f634.PoLC13.NoiseST  seed=f634.PoLC13.NoiseSD
  P : Outport  VectorParamsAs1DForOutWhenUnconnected=off
  wires:
  Sum/1 -> P/1
  noise/1 -> Sum/2
  base/1 -> Sum/1

== system IEEE_13_BUS_Radial/f634/CONTROLLERS/lPoLC14 ==
  Sum : Sum  Inputs=|++
  base : simulink/Sources/Repeating Sequence Stair  OutValues=f634.PoLC14.l  tsamp=f634.PoLC14.ST  OutMin=[]  OutMax=[]  OutDataTypeStr=double  OutputDataTypeScalingMode=double  OutDataType=fixdt(0,8)  ConRadixGroup=Best Precision: Vector-wise  OutScaling=2^-12
  noise : simulink/Sources/Band-Limited White Noise  Cov=f634.PoLC14.Noise  Ts=f634.PoLC14.NoiseST  seed=f634.PoLC14.NoiseSD
  P : Outport  VectorParamsAs1DForOutWhenUnconnected=off
  wires:
  Sum/1 -> P/1
  noise/1 -> Sum/2
  base/1 -> Sum/1

== system IEEE_13_BUS_Radial/f634/CONTROLLERS/lPoLC15 ==
  Sum : Sum  Inputs=|++
  base : simulink/Sources/Repeating Sequence Stair  OutValues=f634.PoLC15.l  tsamp=f634.PoLC15.ST  OutMin=[]  OutMax=[]  OutDataTypeStr=double  OutputDataTypeScalingMode=double  OutDataType=fixdt(0,8)  ConRadixGroup=Best Precision: Vector-wise  OutScaling=2^-12
  noise : simulink/Sources/Band-Limited White Noise  Cov=f634.PoLC15.Noise  Ts=f634.PoLC15.NoiseST  seed=f634.PoLC15.NoiseSD
  P : Outport  VectorParamsAs1DForOutWhenUnconnected=off
  wires:
  Sum/1 -> P/1
  noise/1 -> Sum/2
  base/1 -> Sum/1

== system IEEE_13_BUS_Radial/f634/CONTROLLERS/lPoLC16 ==
  cv : Inport
  Sum : Sum  Inputs=|++
  Terminator : Terminator
  base : simulink/Sources/Repeating Sequence Stair  OutValues=f634.PoLC16.l  tsamp=f634.PoLC16.ST  OutMin=[]  OutMax=[]  OutDataTypeStr=double  OutputDataTypeScalingMode=double  OutDataType=fixdt(0,8)  ConRadixGroup=Best Precision: Vector-wise  OutScaling=2^-12
  noise : simulink/Sources/Band-Limited White Noise  Cov=f634.PoLC16.Noise  Ts=f634.PoLC16.NoiseST  seed=f634.PoLC16.NoiseSD
  P : Outport  VectorParamsAs1DForOutWhenUnconnected=off
  wires:
  Sum/1 -> Terminator/1
  noise/1 -> Sum/2
  base/1 -> Sum/1
  cv/1 -> P/1

== system IEEE_13_BUS_Radial/f634/CONTROLLERS/lPoLC2 ==
  Sum : Sum  Inputs=|++
  base : simulink/Sources/Repeating Sequence Stair  OutValues=f634.PoLC2.l  tsamp=f634.PoLC2.ST  OutMin=[]  OutMax=[]  OutDataTypeStr=double  OutputDataTypeScalingMode=double  OutDataType=fixdt(0,8)  ConRadixGroup=Best Precision: Vector-wise  OutScaling=2^-12
  noise : simulink/Sources/Band-Limited White Noise  Cov=f634.PoLC2.Noise  Ts=f634.PoLC2.NoiseST  seed=f634.PoLC2.NoiseSD
  P : Outport  VectorParamsAs1DForOutWhenUnconnected=off
  wires:
  Sum/1 -> P/1
  noise/1 -> Sum/2
  base/1 -> Sum/1

== system IEEE_13_BUS_Radial/f634/CONTROLLERS/lPoLC3 ==
  Sum : Sum  Inputs=|++
  base : simulink/Sources/Repeating Sequence Stair  OutValues=f634.PoLC3.l  tsamp=f634.PoLC3.ST  OutMin=[]  OutMax=[]  OutDataTypeStr=double  OutputDataTypeScalingMode=double  OutDataType=fixdt(0,8)  ConRadixGroup=Best Precision: Vector-wise  OutScaling=2^-12
  noise : simulink/Sources/Band-Limited White Noise  Cov=f634.PoLC3.Noise  Ts=f634.PoLC3.NoiseST  seed=f634.PoLC3.NoiseSD
  P : Outport  VectorParamsAs1DForOutWhenUnconnected=off
  wires:
  Sum/1 -> P/1
  noise/1 -> Sum/2
  base/1 -> Sum/1

== system IEEE_13_BUS_Radial/f634/CONTROLLERS/lPoLC4 ==
  Sum : Sum  Inputs=|++
  base : simulink/Sources/Repeating Sequence Stair  OutValues=f634.PoLC4.l  tsamp=f634.PoLC4.ST  OutMin=[]  OutMax=[]  OutDataTypeStr=double  OutputDataTypeScalingMode=double  OutDataType=fixdt(0,8)  ConRadixGroup=Best Precision: Vector-wise  OutScaling=2^-12
  noise : simulink/Sources/Band-Limited White Noise  Cov=f634.PoLC4.Noise  Ts=f634.PoLC4.NoiseST  seed=f634.PoLC4.NoiseSD
  P : Outport  VectorParamsAs1DForOutWhenUnconnected=off
  wires:
  Sum/1 -> P/1
  noise/1 -> Sum/2
  base/1 -> Sum/1

== system IEEE_13_BUS_Radial/f634/CONTROLLERS/lPoLC5 ==
  Sum : Sum  Inputs=|++
  base : simulink/Sources/Repeating Sequence Stair  OutValues=f634.PoLC5.l  tsamp=f634.PoLC5.ST  OutMin=[]  OutMax=[]  OutDataTypeStr=double  OutputDataTypeScalingMode=double  OutDataType=fixdt(0,8)  ConRadixGroup=Best Precision: Vector-wise  OutScaling=2^-12
  noise : simulink/Sources/Band-Limited White Noise  Cov=f634.PoLC5.Noise  Ts=f634.PoLC5.NoiseST  seed=f634.PoLC5.NoiseSD
  P : Outport  VectorParamsAs1DForOutWhenUnconnected=off
  wires:
  Sum/1 -> P/1
  noise/1 -> Sum/2
  base/1 -> Sum/1

== system IEEE_13_BUS_Radial/f634/CONTROLLERS/lPoLC6 ==
  Sum : Sum  Inputs=|++
  base : simulink/Sources/Repeating Sequence Stair  OutValues=f634.PoLC6.l  tsamp=f634.PoLC6.ST  OutMin=[]  OutMax=[]  OutDataTypeStr=double  OutputDataTypeScalingMode=double  OutDataType=fixdt(0,8)  ConRadixGroup=Best Precision: Vector-wise  OutScaling=2^-12
  noise : simulink/Sources/Band-Limited White Noise  Cov=f634.PoLC6.Noise  Ts=f634.PoLC6.NoiseST  seed=f634.PoLC6.NoiseSD
  P : Outport  VectorParamsAs1DForOutWhenUnconnected=off
  wires:
  Sum/1 -> P/1
  noise/1 -> Sum/2
  base/1 -> Sum/1

== system IEEE_13_BUS_Radial/f634/CONTROLLERS/lPoLC7 ==
  Sum : Sum  Inputs=|++
  base : simulink/Sources/Repeating Sequence Stair  OutValues=f634.PoLC7.l  tsamp=f634.PoLC7.ST  OutMin=[]  OutMax=[]  OutDataTypeStr=double  OutputDataTypeScalingMode=double  OutDataType=fixdt(0,8)  ConRadixGroup=Best Precision: Vector-wise  OutScaling=2^-12
  noise : simulink/Sources/Band-Limited White Noise  Cov=f634.PoLC7.Noise  Ts=f634.PoLC7.NoiseST  seed=f634.PoLC7.NoiseSD
  P : Outport  VectorParamsAs1DForOutWhenUnconnected=off
  wires:
  Sum/1 -> P/1
  noise/1 -> Sum/2
  base/1 -> Sum/1

== system IEEE_13_BUS_Radial/f634/CONTROLLERS/lPoLC8 ==
  Sum : Sum  Inputs=|++
  base : simulink/Sources/Repeating Sequence Stair  OutValues=f634.PoLC8.l  tsamp=f634.PoLC8.ST  OutMin=[]  OutMax=[]  OutDataTypeStr=double  OutputDataTypeScalingMode=double  OutDataType=fixdt(0,8)  ConRadixGroup=Best Precision: Vector-wise  OutScaling=2^-12
  noise : simulink/Sources/Band-Limited White Noise  Cov=f634.PoLC8.Noise  Ts=f634.PoLC8.NoiseST  seed=f634.PoLC8.NoiseSD
  P : Outport  VectorParamsAs1DForOutWhenUnconnected=off
  wires:
  Sum/1 -> P/1
  noise/1 -> Sum/2
  base/1 -> Sum/1

== system IEEE_13_BUS_Radial/f634/CONTROLLERS/lPoLC9 ==
  Sum : Sum  Inputs=|++
  base : simulink/Sources/Repeating Sequence Stair  OutValues=f634.PoLC9.l  tsamp=f634.PoLC9.ST  OutMin=[]  OutMax=[]  OutDataTypeStr=double  OutputDataTypeScalingMode=double  OutDataType=fixdt(0,8)  ConRadixGroup=Best Precision: Vector-wise  OutScaling=2^-12
  noise : simulink/Sources/Band-Limited White Noise  Cov=f634.PoLC9.Noise  Ts=f634.PoLC9.NoiseST  seed=f634.PoLC9.NoiseSD
  P : Outport  VectorParamsAs1DForOutWhenUnconnected=off
  wires:
  Sum/1 -> P/1
  noise/1 -> Sum/2
  base/1 -> Sum/1

== system IEEE_13_BUS_Radial/f634/OPERATIONS GATEWAY/Agent Communications ==
  Enable : EnablePort
  Constant : Constant  Value=0
  Out1 : Outport  VectorParamsAs1DForOutWhenUnconnected=off
  wires:
  Constant/1 -> Out1/1

== system IEEE_13_BUS_Radial/f645/CONTROLLERS/lPoLC1 ==
  Sum : Sum  Inputs=|++
  base : simulink/Sources/Repeating Sequence Stair  OutValues=f645.PoLC1.l  tsamp=f645.PoLC1.ST  OutMin=[]  OutMax=[]  OutDataTypeStr=double  OutputDataTypeScalingMode=double  OutDataType=fixdt(0,8)  ConRadixGroup=Best Precision: Vector-wise  OutScaling=2^-12
  noise : simulink/Sources/Band-Limited White Noise  Cov=f645.PoLC1.Noise  Ts=f645.PoLC1.NoiseST  seed=f645.PoLC1.NoiseSD
  P : Outport  VectorParamsAs1DForOutWhenUnconnected=off
  wires:
  Sum/1 -> P/1
  noise/1 -> Sum/2
  base/1 -> Sum/1

== system IEEE_13_BUS_Radial/f645/CONTROLLERS/lPoLC10 ==
  Sum : Sum  Inputs=|++
  base : simulink/Sources/Repeating Sequence Stair  OutValues=f645.PoLC10.l  tsamp=f645.PoLC10.ST  OutMin=[]  OutMax=[]  OutDataTypeStr=double  OutputDataTypeScalingMode=double  OutDataType=fixdt(0,8)  ConRadixGroup=Best Precision: Vector-wise  OutScaling=2^-12
  noise : simulink/Sources/Band-Limited White Noise  Cov=f645.PoLC10.Noise  Ts=f645.PoLC10.NoiseST  seed=f645.PoLC10.NoiseSD
  P : Outport  VectorParamsAs1DForOutWhenUnconnected=off
  wires:
  Sum/1 -> P/1
  noise/1 -> Sum/2
  base/1 -> Sum/1

== system IEEE_13_BUS_Radial/f645/CONTROLLERS/lPoLC11 ==
  Sum : Sum  Inputs=|++
  base : simulink/Sources/Repeating Sequence Stair  OutValues=f645.PoLC11.l  tsamp=f645.PoLC11.ST  OutMin=[]  OutMax=[]  OutDataTypeStr=double  OutputDataTypeScalingMode=double  OutDataType=fixdt(0,8)  ConRadixGroup=Best Precision: Vector-wise  OutScaling=2^-12
  noise : simulink/Sources/Band-Limited White Noise  Cov=f645.PoLC11.Noise  Ts=f645.PoLC11.NoiseST  seed=f645.PoLC11.NoiseSD
  P : Outport  VectorParamsAs1DForOutWhenUnconnected=off
  wires:
  Sum/1 -> P/1
  noise/1 -> Sum/2
  base/1 -> Sum/1

== system IEEE_13_BUS_Radial/f645/CONTROLLERS/lPoLC12 ==
  Sum : Sum  Inputs=|++
  base : simulink/Sources/Repeating Sequence Stair  OutValues=f645.PoLC12.l  tsamp=f645.PoLC12.ST  OutMin=[]  OutMax=[]  OutDataTypeStr=double  OutputDataTypeScalingMode=double  OutDataType=fixdt(0,8)  ConRadixGroup=Best Precision: Vector-wise  OutScaling=2^-12
  noise : simulink/Sources/Band-Limited White Noise  Cov=f645.PoLC12.Noise  Ts=f645.PoLC12.NoiseST  seed=f645.PoLC12.NoiseSD
  P : Outport  VectorParamsAs1DForOutWhenUnconnected=off
  wires:
  Sum/1 -> P/1
  noise/1 -> Sum/2
  base/1 -> Sum/1

== system IEEE_13_BUS_Radial/f645/CONTROLLERS/lPoLC13 ==
  Sum : Sum  Inputs=|++
  base : simulink/Sources/Repeating Sequence Stair  OutValues=f645.PoLC13.l  tsamp=f645.PoLC13.ST  OutMin=[]  OutMax=[]  OutDataTypeStr=double  OutputDataTypeScalingMode=double  OutDataType=fixdt(0,8)  ConRadixGroup=Best Precision: Vector-wise  OutScaling=2^-12
  noise : simulink/Sources/Band-Limited White Noise  Cov=f645.PoLC13.Noise  Ts=f645.PoLC13.NoiseST  seed=f645.PoLC13.NoiseSD
  P : Outport  VectorParamsAs1DForOutWhenUnconnected=off
  wires:
  Sum/1 -> P/1
  noise/1 -> Sum/2
  base/1 -> Sum/1

== system IEEE_13_BUS_Radial/f645/CONTROLLERS/lPoLC14 ==
  Sum : Sum  Inputs=|++
  base : simulink/Sources/Repeating Sequence Stair  OutValues=f645.PoLC14.l  tsamp=f645.PoLC14.ST  OutMin=[]  OutMax=[]  OutDataTypeStr=double  OutputDataTypeScalingMode=double  OutDataType=fixdt(0,8)  ConRadixGroup=Best Precision: Vector-wise  OutScaling=2^-12
  noise : simulink/Sources/Band-Limited White Noise  Cov=f645.PoLC14.Noise  Ts=f645.PoLC14.NoiseST  seed=f645.PoLC14.NoiseSD
  P : Outport  VectorParamsAs1DForOutWhenUnconnected=off
  wires:
  Sum/1 -> P/1
  noise/1 -> Sum/2
  base/1 -> Sum/1
